simulink model "modeleetat"  (R2020a)
settings: Solver=VariableStepAuto  StartTime=0.0  StopTime=30  RelTol=1e-3
values from neighbouring files (symbols this model uses):
  A = [0 1 ... (first row only)    [identificat.m]    (also in projet.mat = [0  1; 0  0])
  B = K_pos*[0 ... (first row only)    [identificat.m]    (also in projet.mat = [0 0.907])
  K = place(A,B,paul)    [identificat.m]    (also in projet.mat = [0.286659316428 0.220507166483])
libraries: cstblocks x1
settings Model: Creator=soual  LastModifiedBy=soual

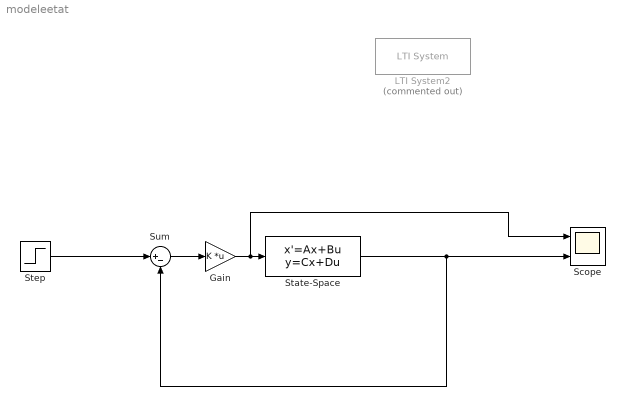
== system modeleetat ==
  Gain : Gain  Gain=K  Multiplication=Matrix(K*u)
  LTI System2 : cstblocks/LTI System  Commented=on  sys=TF  IC=[]
  Scope : Scope  NumInputPorts=2
  State-Space : StateSpace  A=A  B=B  C=[1 0; 0 1]  D=[0;0]  InitialCondition=0
  Step : Step  Time=5  After=2  SampleTime=0
  Sum : Sum  Inputs=|+-
  wires:
  Step/1 -> Sum/1
  Sum/1 -> Gain/1
  State-Space/1 -> Sum/2, Scope/2
  Gain/1 -> Scope/1, State-Space/1
